simulink model "LEGO_ServoMotor"  (R2014a)
settings: Solver=ode3  SolverMode=SingleTasking  StartTime=0.0  StopTime=30  FixedStep=ts1  RelTol=1e-3
InitFcn:
  | ts1 = 0.004;
  | Ts = 0.04;
  | f = 0.25;
  | kp = 0.0279;
  | ki = 0.0403;
libraries: legonxtlib x8, simulink x2
CloseFcn:
  | clear ts1,Ts,kp,ki,f;
settings Model: ExtModeTrigDuration=2  Creator=Alphonso Monk  LastModifiedBy=Alphonso Monk
settings OptimizationCC: OptimizeModelRefInitCode=on  LifeSpan=1
settings DebuggingCC: UnderspecifiedInitializationDetection=Classic  SolverPrmCheckMsg=none
settings HardwareCC: ProdLargestAtomicInteger=Long  ProdLargestAtomicFloat=Float  ProdEndianess=LittleEndian  ProdHWDeviceType=ARM Compatible->ARM 7
settings RTWCC: SystemTargetFile=realtime.tlc  GenerateMakefile=off  TemplateMakefile=realtime.tmf  Description=Run on Target Hardware  RTWVerbose=off  ProcessScript=realtime_make_rtw_hook
settings STFCustomTargetCC: TargetLibSuffix=.a  GenerateSampleERTMain=on  ConcurrentExecutionCompliant=off  GeneratePreprocessorConditionals=Use local settings  ERTCustomFileBanners=on  SupportNonInlinedSFcns=off  SupportVariableSizeSignals=on  MATLABClassNameForMDSCustomization=Simulink.SoftwareTarget.ERTCustomization  GRTInterface=off  SystemTargetFile=realtime.tlc
settings ERTTargetCC: CombineOutputUpdateFcns=off  SupportContinuousTime=on  SupportVariableSizeSignals=on  ExtModeTransport=2  ExtModeMexFile=ext_serial_win32_comm_no_acks_rtt  ExtModeMexArgs=0 1 9600  ERTSrcFileBannerTemplate=realtime_code_template.cgt  ERTHdrFileBannerTemplate=realtime_code_template.cgt  ERTDataSrcFileTemplate=realtime_code_template.cgt  ERTDataHdrFileTemplate=realtime_code_template.cgt  ERTCustomFileTemplate=realtime_file_process.tlc

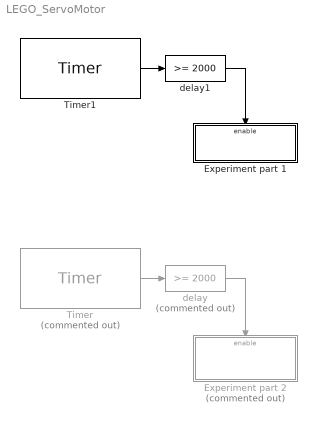
== system LEGO_ServoMotor ==
  Experiment part 1 : Subsystem
  Experiment part 2 : Subsystem  Commented=on  TreatAsAtomicUnit=on
  Timer : legonxtlib/Timer  Commented=on  sampleTime=0.1
  Timer1 : legonxtlib/Timer  sampleTime=0.1
  delay : simulink/Logic and Bit Operations/Compare To Constant  Commented=on  relop=>=  const=2000  OutDataTypeStr=boolean
  delay1 : simulink/Logic and Bit Operations/Compare To Constant  relop=>=  const=2000  OutDataTypeStr=boolean
  wires:
  Timer/1 -> delay/1
  delay/1 -> Experiment part 2/Enable
  Timer1/1 -> delay1/1
  delay1/1 -> Experiment part 1/Enable

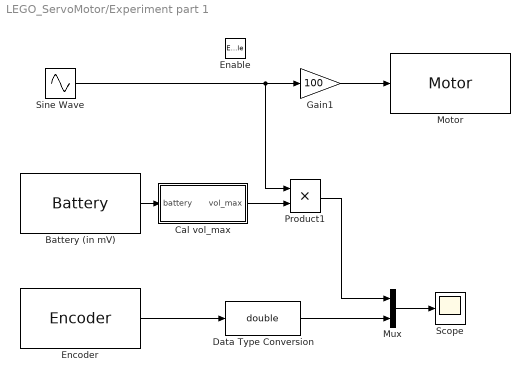
== system LEGO_ServoMotor/Experiment part 1 ==
  Enable : EnablePort
  Battery (in mV) : legonxtlib/Battery  sampleTime=Ts
  Cal vol_max : Subsystem
  Data Type Conversion : DataTypeConversion  OutDataTypeStr=double
  Encoder : legonxtlib/Encoder  portNumber=A  opMode=No reset  sampleTime=ts1
  Gain1 : Gain  Gain=100
  Motor : legonxtlib/Motor  sportNumber=A  sstopAction=Brake
  Mux : Mux  Inputs=2
  Product1 : Product  Inputs=**
  Scope : Scope
      settings: YMin=-50  YMax=275  SaveName=motorResponse
  Sine Wave : Sin  Frequency=2*pi*f  SampleTime=ts1  VectorParams1D=off
  wires:
  Encoder/1 -> Data Type Conversion/1
  Mux/1 -> Scope/1
  Sine Wave/1 -> Gain1/1, Product1/1
  Battery (in mV)/1 -> Cal vol_max/1(battery)
  Cal vol_max/1(vol_max) -> Product1/2
  Product1/1 -> Mux/1
  Data Type Conversion/1 -> Mux/2
  Gain1/1 -> Motor/1

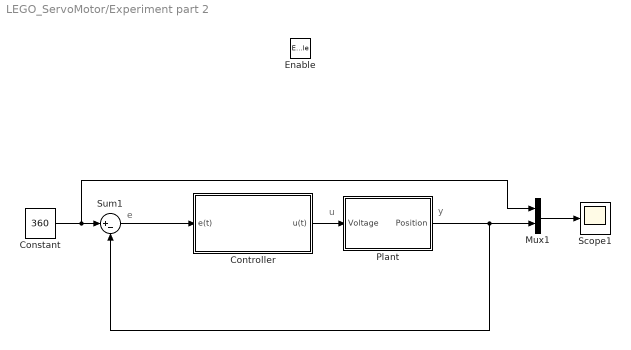
== system LEGO_ServoMotor/Experiment part 2 ==
  note: e
  note: u
  note: y
  Enable : EnablePort
  Constant : Constant  Value=360
  Controller : Subsystem
  Mux1 : Mux  Inputs=2
  Plant : Subsystem
  Scope1 : Scope
      settings: TimeRange=10  YMin=0  YMax=475  SaveName=motorResponse1
  Sum1 : Sum  Inputs=|+-
  wires:
  Plant/1(Position) -> Sum1/2, Mux1/2
  Mux1/1 -> Scope1/1
  Constant/1 -> Mux1/1, Sum1/1
  Controller/1(u(t)) -> Plant/1(Voltage)
  Sum1/1 -> Controller/1(e(t))

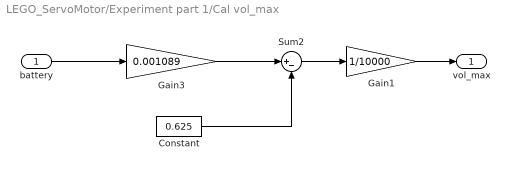
== system LEGO_ServoMotor/Experiment part 1/Cal vol_max ==
  battery : Inport
  Constant : Constant  Value=0.625  OutDataTypeStr=single
      settings: AttributesFormatString=DataType = %<OutDataTypeStr>
  Gain1 : Gain  Gain=1/10000
  Gain3 : Gain  Gain=0.001089  OutDataTypeStr=Inherit: Same as input  ParamDataTypeStr=Inherit: Same as input
  Sum2 : Sum  Inputs=|+-  OutDataTypeStr=Inherit: Same as first input
  vol_max : Outport
  wires:
  Gain3/1 -> Sum2/1
  Sum2/1 -> Gain1/1
  Constant/1 -> Sum2/2
  battery/1 -> Gain3/1
  Gain1/1 -> vol_max/1

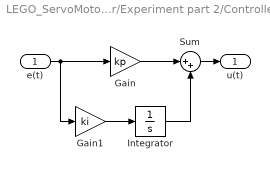
== system LEGO_ServoMotor/Experiment part 2/Controller ==
  e(t) : Inport
  Gain : Gain  Gain=kp
  Gain1 : Gain  Gain=ki
  Integrator : Integrator
  Sum : Sum  Inputs=|++
  u(t) : Outport
  wires:
  Integrator/1 -> Sum/2
  Gain1/1 -> Integrator/1
  Gain/1 -> Sum/1
  e(t)/1 -> Gain1/1, Gain/1
  Sum/1 -> u(t)/1

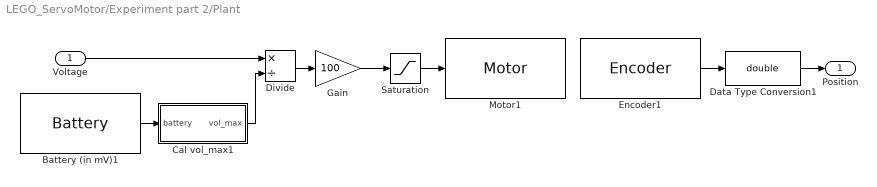
== system LEGO_ServoMotor/Experiment part 2/Plant ==
  Voltage : Inport
  Battery (in mV)1 : legonxtlib/Battery  sampleTime=Ts
  Cal vol_max1 : Subsystem
  Data Type Conversion1 : DataTypeConversion  OutDataTypeStr=double
  Divide : Product  Inputs=*/
  Encoder1 : legonxtlib/Encoder  portNumber=A  opMode=No reset  sampleTime=ts1
  Gain : Gain  Gain=100
  Motor1 : legonxtlib/Motor  sportNumber=A  sstopAction=Brake
  Saturation : Saturate  UpperLimit=100  LowerLimit=-100
  Position : Outport
  wires:
  Saturation/1 -> Motor1/1
  Encoder1/1 -> Data Type Conversion1/1
  Data Type Conversion1/1 -> Position/1
  Voltage/1 -> Divide/1
  Battery (in mV)1/1 -> Cal vol_max1/1(battery)
  Cal vol_max1/1(vol_max) -> Divide/2
  Divide/1 -> Gain/1
  Gain/1 -> Saturation/1

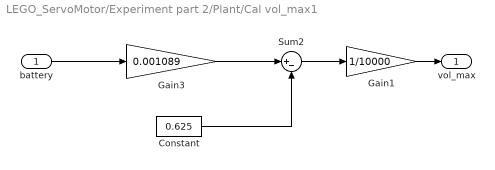
== system LEGO_ServoMotor/Experiment part 2/Plant/Cal vol_max1 ==
  battery : Inport
  Constant : Constant  Value=0.625  OutDataTypeStr=single
      settings: AttributesFormatString=DataType = %<OutDataTypeStr>
  Gain1 : Gain  Gain=1/10000
  Gain3 : Gain  Gain=0.001089  OutDataTypeStr=Inherit: Same as input  ParamDataTypeStr=Inherit: Same as input
  Sum2 : Sum  Inputs=|+-  OutDataTypeStr=Inherit: Same as first input
  vol_max : Outport
  wires:
  Gain1/1 -> vol_max/1
  battery/1 -> Gain3/1
  Constant/1 -> Sum2/2
  Sum2/1 -> Gain1/1
  Gain3/1 -> Sum2/1
